simulink model "partB_sim"  (R2021b)
settings: Solver=FixedStepAuto  StartTime=0.0  StopTime=30  FixedStep=0.01  RelTol=1e-3
values from neighbouring files (symbols this model uses):
  Kd_g = 0.335    [lab2.m]
  Ki_g = 0.05    [lab2.m]
  Kp_g = 3.355    [lab2.m]
libraries: simulink x1
settings Model: Creator=DSDLn  LastModifiedBy=DSDLn

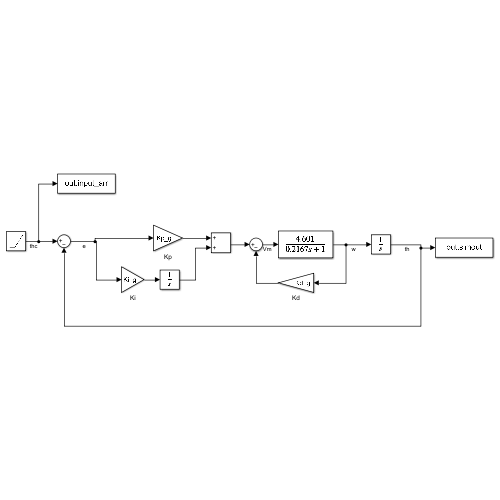
[thumbnail: Simulink's stored preview of the top-level diagram]
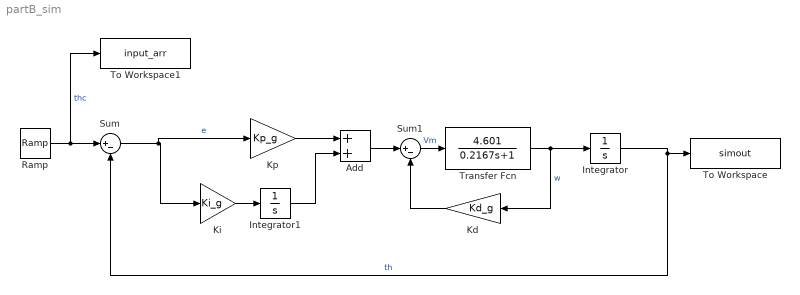
== system partB_sim ==
  Add : Sum
  Integrator : Integrator
  Integrator1 : Integrator
  Kd : Gain  Gain=Kd_g
  Ki : Gain  Gain=Ki_g
  Kp : Gain  Gain=Kp_g
  Ramp : simulink/Sources/Ramp  slope=1  start=0  InitialOutput=0
  Sum : Sum  Inputs=|+-
  Sum1 : Sum  Inputs=|+-
  To Workspace : ToWorkspace  VariableName=simout  SampleTime=-1
  To Workspace1 : ToWorkspace  VariableName=input_arr  SampleTime=-1
  Transfer Fcn : TransferFcn  Numerator=[4.601]  Denominator=[0.2167 1]
  wires:
  Ki/1 -> Integrator1/1
  Integrator1/1 -> Add/2
  Kp/1 -> Add/1
  Sum/1 -> Ki/1, Kp/1  "e"
  Integrator/1 -> Sum/2, To Workspace/1  "th"
  Add/1 -> Sum1/1
  Sum1/1 -> Transfer Fcn/1  "Vm"
  Transfer Fcn/1 -> Kd/1, Integrator/1  "w"
  Kd/1 -> Sum1/2
  Ramp/1 -> To Workspace1/1, Sum/1  "thc"
